simulink model "filterdesign"  (R2020a)
settings: Solver=VariableStepAuto  StartTime=0.0  StopTime=10.0  RelTol=1e-3
settings Model: Creator=Hp  LastModifiedBy=Hp

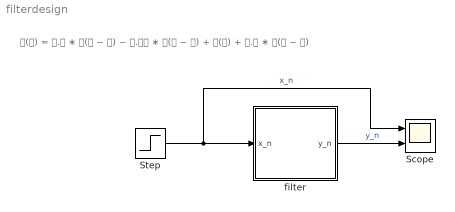
== system filterdesign ==
  note: 𝐲(𝐧) = 𝟎.𝟓 ∗ 𝐲(𝐧 − 𝟏) − 𝟎.𝟐𝟓 ∗ 𝐲(𝐧 − 𝟐) + 𝐱(𝐧) + 𝟎.𝟒 ∗ 𝐱(𝐧 − 𝟏)
  Scope : Scope  NumInputPorts=2
  Step : Step  SampleTime=0.001
  filter : Subsystem
  wires:
  Step/1 -> filter/1(x_n), Scope/1  "x_n"
  filter/1(y_n) -> Scope/2  "y_n"

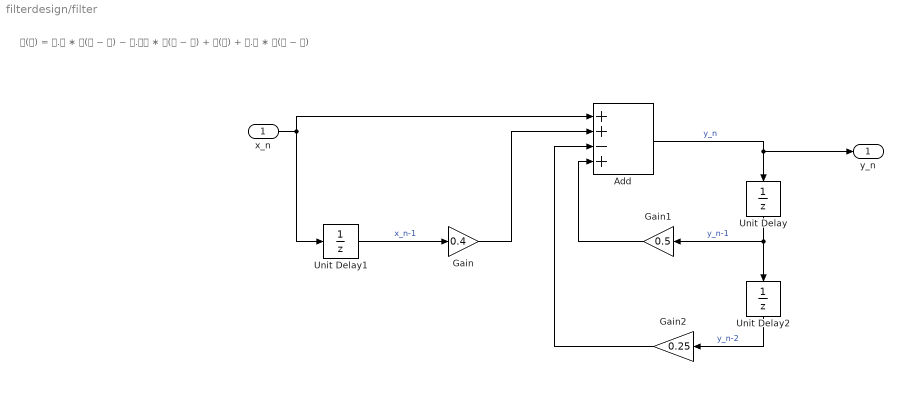
== system filterdesign/filter ==
  note: 𝐲(𝐧) = 𝟎.𝟓 ∗ 𝐲(𝐧 − 𝟏) − 𝟎.𝟐𝟓 ∗ 𝐲(𝐧 − 𝟐) + 𝐱(𝐧) + 𝟎.𝟒 ∗ 𝐱(𝐧 − 𝟏)
  x_n : Inport
  Add : Sum  Inputs=++-+
  Gain : Gain  Gain=0.4
  Gain1 : Gain  Gain=0.5
  Gain2 : Gain  Gain=0.25
  Unit Delay : UnitDelay  SampleTime=-1  HasFrameUpgradeWarning=on
  Unit Delay1 : UnitDelay  SampleTime=-1  HasFrameUpgradeWarning=on
  Unit Delay2 : UnitDelay  SampleTime=-1  HasFrameUpgradeWarning=on
  y_n : Outport
  wires:
  Gain1/1 -> Add/4
  Unit Delay1/1 -> Gain/1  "x_n-1"
  Gain2/1 -> Add/3
  Unit Delay2/1 -> Gain2/1  "y_n-2"
  Gain/1 -> Add/2
  Unit Delay/1 -> Unit Delay2/1, Gain1/1  "y_n-1"
  Add/1 -> y_n/1, Unit Delay/1  "y_n"
  x_n/1 -> Add/1, Unit Delay1/1
